simulink model "SimulinkOminidirectinalDrone"  (R2025a)
settings: Solver=ode15s  StartTime=0.0  StopTime=10  RelTol=1e-4
values from neighbouring files (symbols this model uses):
  AUM = 3.057    [Parameter.m]
  Cq = 0.013    [Parameter.m]
  Ct = 0.013    [Parameter.m]
  g = 9.8    [Parameter.m]
  H = 0.05    [Parameter.m]
  Ixx = 0.49827    [Parameter.m]
  Iyy = 0.48993    [Parameter.m]
  Izz = 0.82777    [Parameter.m]
  L = 0.25    [Parameter.m]
  R_rad = 0.15    [Parameter.m]
  rho = 1.18195    [Parameter.m]
  W = diag([0.994, 0.003, 0.003, 0.994, 0.003, 0.003,            0.994, 0.003, 0.003, 0.994, 0.003, 0.003])    [Parameter.m]
libraries: sharedutil x4, aerolibobsolete x1
(part 1 of 2)
settings Model: Creator=Nguyen_Duc  LastModifiedBy=Nguyen_Duc
settings RTWCC: GPUComputeCapability=3.5

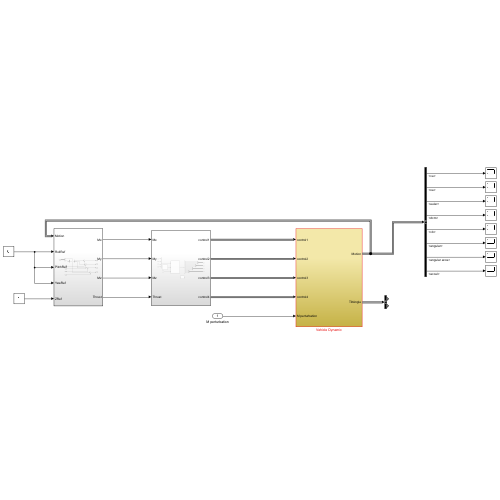
[thumbnail: Simulink's stored preview of the top-level diagram]
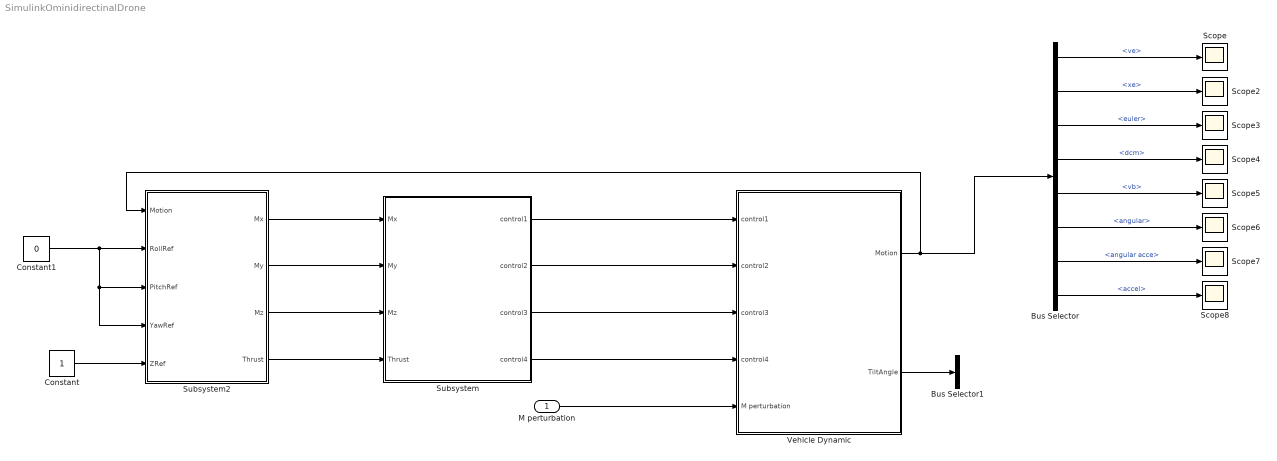
== system SimulinkOminidirectinalDrone ==
  M perturbation : Inport
  Bus Selector : BusSelector  OutputSignals=ve,xe,euler,dcm,vb,angular,angular acce,accel
  Bus Selector1 : BusSelector  OutputSignals=signal1,signal2
  Constant : Constant
  Constant1 : Constant  Value=0
  Scope{,2..8} (8 alike) : Scope
      Scope settings: ActiveDisplayYMinimum=-12.600361564793616  ActiveDisplayYMaximum=158.14211469770717
      Scope2 settings: ActiveDisplayYMinimum=-253.65470239682742  ActiveDisplayYMaximum=2044.3378889341363  DataLoggingVariableName=ScopeData2
      Scope3 settings: ActiveDisplayYMinimum=-3.8093227520417652  ActiveDisplayYMaximum=3.6702175311661223  DataLoggingVariableName=ScopeData3
      Scope4 settings: ActiveDisplayYMinimum=-1.6887966568785009  ActiveDisplayYMaximum=1.3036985575111188  DataLoggingVariableName=ScopeData4
      Scope5 settings: ActiveDisplayYMinimum=-51.9670542151825  ActiveDisplayYMaximum=175.32388672860668  DataLoggingVariableName=ScopeData5
      Scope6 settings: ActiveDisplayYMinimum=-1  ActiveDisplayYMaximum=1  DataLoggingVariableName=ScopeData6
      Scope7 settings: DataLoggingVariableName=ScopeData7
      Scope8 settings: DataLoggingVariableName=ScopeData8
  Subsystem : Subsystem
  Subsystem2 : Subsystem
  Vehicle Dynamic : Subsystem
  wires:
  Subsystem/1(control1) -> Vehicle Dynamic/1(control1)
  Subsystem/2(control2) -> Vehicle Dynamic/2(control2)
  Subsystem/3(control3) -> Vehicle Dynamic/3(control3)
  Subsystem/4(control4) -> Vehicle Dynamic/4(control4)
  M perturbation/1 -> Vehicle Dynamic/5(M perturbation)
  Vehicle Dynamic/2(TiltAngle) -> Bus Selector1/1
  Vehicle Dynamic/1(Motion) -> Bus Selector/1, Subsystem2/1(Motion)
  Bus Selector/1 -> Scope/1  "<ve>"
  Bus Selector/2 -> Scope2/1  "<xe>"
  Bus Selector/3 -> Scope3/1  "<euler>"
  Bus Selector/4 -> Scope4/1  "<dcm>"
  Bus Selector/5 -> Scope5/1  "<vb>"
  Bus Selector/6 -> Scope6/1  "<angular>"
  Bus Selector/7 -> Scope7/1  "<angular acce>"
  Bus Selector/8 -> Scope8/1  "<accel>"
  Constant/1 -> Subsystem2/5(ZRef)
  Constant1/1 -> Subsystem2/4(YawRef), Subsystem2/3(PitchRef), Subsystem2/2(RollRef)
  Subsystem2/1(Mx) -> Subsystem/1(Mx)
  Subsystem2/2(My) -> Subsystem/2(My)
  Subsystem2/3(Mz) -> Subsystem/3(Mz)
  Subsystem2/4(Thrust) -> Subsystem/4(Thrust)

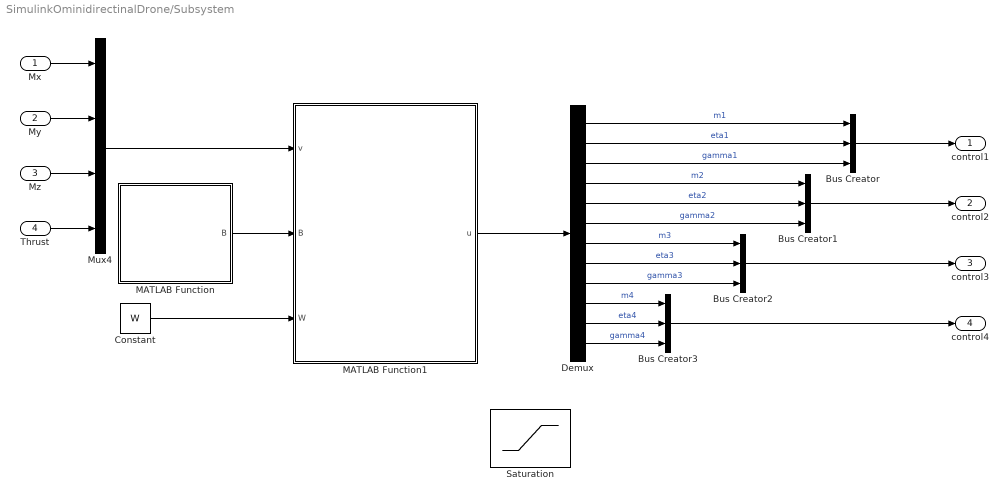
== system SimulinkOminidirectinalDrone/Subsystem ==
  Mx : Inport
  My : Inport  Port=2
  Mz : Inport  Port=3
  Thrust : Inport  Port=4
  Bus Creator{,1..3} (4 alike) : BusCreator  Inputs=3
  Constant : Constant  Value=W
  Demux : Demux  Outputs=12
  MATLAB Function : MATLAB Function  TreatAsAtomicUnit=on
  MATLAB Function1 : MATLAB Function  TreatAsAtomicUnit=on
  Mux4 : Mux
  Saturation : Saturate  UpperLimit="[1  30*pi/180  0.2  1  30*pi/180  0.2  1  30*pi/180  0.2  1  30*pi/180  0.2]"  LowerLimit="[0 -30*pi/180 -0.2  0 -30*pi/180 -0.2  0 -30*pi/180 -0.2  0 -30*pi/180 -0.2]"
  control1 : Outport
  control2 : Outport  Port=2
  control3 : Outport  Port=3
  control4 : Outport  Port=4
  wires:
  MATLAB Function/1(B) -> MATLAB Function1/2(B)
  Mux4/1 -> MATLAB Function1/1(v)
  Demux/1 -> Bus Creator/1  "m1"
  Bus Creator/1 -> control1/1
  Demux/3 -> Bus Creator/3  "gamma1"
  Demux/2 -> Bus Creator/2  "eta1"
  Demux/4 -> Bus Creator1/1  "m2"
  Demux/5 -> Bus Creator1/2  "eta2"
  Demux/6 -> Bus Creator1/3  "gamma2"
  Demux/7 -> Bus Creator2/1  "m3"
  Demux/8 -> Bus Creator2/2  "eta3"
  Demux/9 -> Bus Creator2/3  "gamma3"
  Demux/10 -> Bus Creator3/1  "m4"
  Demux/11 -> Bus Creator3/2  "eta4"
  Demux/12 -> Bus Creator3/3  "gamma4"
  Bus Creator1/1 -> control2/1
  Bus Creator2/1 -> control3/1
  Bus Creator3/1 -> control4/1
  Mx/1 -> Mux4/1
  My/1 -> Mux4/2
  Mz/1 -> Mux4/3
  Thrust/1 -> Mux4/4
  Constant/1 -> MATLAB Function1/3(W)
  MATLAB Function1/1(u) -> Demux/1

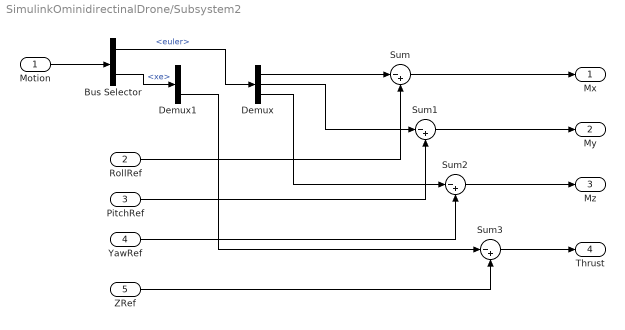
== system SimulinkOminidirectinalDrone/Subsystem2 ==
  Motion : Inport
  RollRef : Inport  Port=2
  PitchRef : Inport  Port=3
  YawRef : Inport  Port=4
  ZRef : Inport  Port=5
  Bus Selector : BusSelector  OutputSignals=euler,xe
  Demux : Demux  Outputs=3
  Demux1 : Demux  Outputs=3
  Sum{,1..3} (4 alike) : Sum  Inputs=|-+
  Mx : Outport
  My : Outport  Port=2
  Mz : Outport  Port=3
  Thrust : Outport  Port=4
  wires:
  Motion/1 -> Bus Selector/1
  Bus Selector/1 -> Demux/1  "<euler>"
  Demux/1 -> Sum/1
  RollRef/1 -> Sum/2
  Sum/1 -> Mx/1
  PitchRef/1 -> Sum1/2
  Sum1/1 -> My/1
  Demux/2 -> Sum1/1
  Sum2/1 -> Mz/1
  Demux/3 -> Sum2/1
  YawRef/1 -> Sum2/2
  Bus Selector/2 -> Demux1/1  "<xe>"
  Sum3/1 -> Thrust/1
  Demux1/3 -> Sum3/1
  ZRef/1 -> Sum3/2

== system SimulinkOminidirectinalDrone/Vehicle Dynamic ==
  control1 : Inport
  control2 : Inport  Port=2
  control3 : Inport  Port=3
  control4 : Inport  Port=4
  M perturbation : Inport  Port=5
  6DOF (Euler Angles) : aerolibobsolete/6DOF (Euler Angles)  units=Metric (MKS)  mtype=Fixed  rep=Euler Angles  xme_0=[0 0 0]  Vm_0=[0 0 0]  eul_0=[0 0 0]  pm_0=[0 0 0]  mass_0=AUM  mass_e=0.5  mass_f=2.0  inertia=[0.49827 0 0; 0 0.48993 0; 0 0 0.82777]  inertia_e=eye(3)  inertia_f=2*eye(3)  k_quat=1.0  vre_flag=on  abi_flag=off  aMode=0  xme_statename=''  Vm_statename=''  eul_statename=''  quat_statename=''  pm_statename=''  mass_statename=''
  Bus Creator : BusCreator  Inputs=8
  Constant : Constant  Value=[0 0 g*AUM]'
  Matrix Multiply : Product  Multiplication=Matrix(*)
  Subsystem1 : Subsystem
  Sum : Sum  Inputs=++|
  Sum1 : Sum  Inputs=|++
  actuator : Subsystem
  Motion : Outport
  TiltAngle : Outport  Port=2
  wires:
  control3/1 -> actuator/4(control3)
  M perturbation/1 -> Sum1/2
  Matrix Multiply/1 -> Sum/1
  6DOF (Euler Angles)/7 -> Bus Creator/7, Subsystem1/2(omegadot)  "angular acce"
  6DOF (Euler Angles)/3 -> Bus Creator/3  "euler"
  Bus Creator/1 -> Motion/1
  control1/1 -> actuator/2(control1)
  6DOF (Euler Angles)/2 -> Bus Creator/2  "xe"
  6DOF (Euler Angles)/1 -> Bus Creator/1  "ve"
  control2/1 -> actuator/3(control2)
  control4/1 -> actuator/5(control4)
  Constant/1 -> Matrix Multiply/2
  6DOF (Euler Angles)/8 -> Bus Creator/8  "accel"
  6DOF (Euler Angles)/6 -> Subsystem1/1(omega), Bus Creator/6  "angular"
  6DOF (Euler Angles)/5 -> Bus Creator/5  "vb"
  6DOF (Euler Angles)/4 -> Matrix Multiply/1, Bus Creator/4  "dcm"
  actuator/3(TiltAngle) -> TiltAngle/1
  Subsystem1/1(Rotation) -> actuator/1(rotation)
  Sum/1 -> 6DOF (Euler Angles)/1
  actuator/1(Forces) -> Sum/2
  actuator/2(Moments) -> Sum1/1
  Sum1/1 -> 6DOF (Euler Angles)/2

== system SimulinkOminidirectinalDrone/Vehicle Dynamic/Subsystem1 ==
  omega : Inport
  omegadot : Inport  Port=2
  Bus Creator : BusCreator  Inputs=6
  Delay : Delay
  Delay1 : Delay
  Delay2 : Delay
  Demux : Demux  Outputs=3
  Demux1 : Demux  Outputs=3
  Rotation : Outport
  wires:
  omega/1 -> Demux/1
  omegadot/1 -> Demux1/1
  Bus Creator/1 -> Rotation/1
  Demux/1 -> Bus Creator/1  "p"
  Demux/2 -> Bus Creator/2  "q"
  Demux/3 -> Bus Creator/3  "r"
  Delay/1 -> Bus Creator/4  "pdot"
  Delay2/1 -> Bus Creator/6  "rdot"
  Delay1/1 -> Bus Creator/5  "qdot"
  Demux1/1 -> Delay/1  "pdot"
  Demux1/2 -> Delay1/1  "qdot"
  Demux1/3 -> Delay2/1  "rdot"

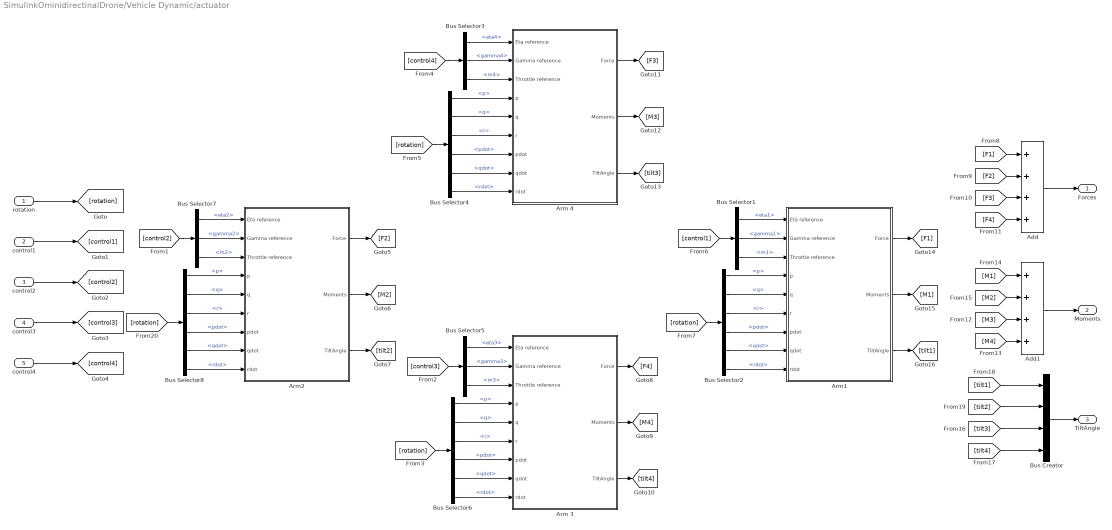
== system SimulinkOminidirectinalDrone/Vehicle Dynamic/actuator ==
  rotation : Inport
  control1 : Inport  Port=2
  control2 : Inport  Port=3
  control3 : Inport  Port=4
  control4 : Inport  Port=5
  Add : Sum  Inputs=++++
  Add1 : Sum  Inputs=++++
  Arm 3 : Subsystem
  Arm 4 : Subsystem
  Arm1 : Subsystem
  Arm2 : Subsystem
  Bus Creator : BusCreator  Inputs=4
  Bus Selector1 : BusSelector  OutputSignals=eta1,gamma1,m1
  Bus Selector{2,4,6,8} (4 alike) : BusSelector  OutputSignals=p,q,r,pdot,qdot,rdot
  Bus Selector3 : BusSelector  OutputSignals=eta4,gamma4,m4
  Bus Selector5 : BusSelector  OutputSignals=eta3,gamma3,m3
  Bus Selector7 : BusSelector  OutputSignals=eta2,gamma2,m2
  Forces : Outport
  Moments : Outport  Port=2
  TiltAngle : Outport  Port=3
  wires:
  control3/1 -> [control3]
  Add/1 -> Forces/1
  [F4] -> Add/4
  Arm1/3(TiltAngle) -> [tilt1]
  [M3] -> Add1/3
  [control1] -> Bus Selector1/1
  Arm1/2(Moments) -> [M1]
  Arm 4/1(Force) -> [F3]
  Bus Selector2/3 -> Arm1/6(r)  "<r>"
  [M2] -> Add1/2
  Arm2/1(Force) -> [F2]
  Arm1/1(Force) -> [F1]
  [M1] -> Add1/1
  [M4] -> Add1/4
  Add1/1 -> Moments/1
  Arm 3/1(Force) -> [F4]
  Bus Selector2/2 -> Arm1/5(q)  "<q>"
  Arm 4/2(Moments) -> [M3]
  Arm 3/2(Moments) -> [M4]
  control1/1 -> [control1]
  Arm2/3(TiltAngle) -> [tilt2]
  Arm 3/3(TiltAngle) -> [tilt4]
  control2/1 -> [control2]
  Bus Selector2/1 -> Arm1/4(p)  "<p>"
  Arm2/2(Moments) -> [M2]
  Arm 4/3(TiltAngle) -> [tilt3]
  rotation/1 -> [rotation]
  control4/1 -> [control4]
  [F3] -> Add/3
  [F1] -> Add/1
  [F2] -> Add/2
  [tilt1] -> Bus Creator/1
  [tilt2] -> Bus Creator/2
  [tilt3] -> Bus Creator/3
  [tilt4] -> Bus Creator/4
  Bus Creator/1 -> TiltAngle/1
  [rotation] -> Bus Selector2/1
  Bus Selector1/1 -> Arm1/1(Eta reference)  "<eta1>"
  Bus Selector1/2 -> Arm1/2(Gamma reference)  "<gamma1>"
  Bus Selector1/3 -> Arm1/3(Throttle reference)  "<m1>"
  Bus Selector2/4 -> Arm1/7(pdot)  "<pdot>"
  [control4] -> Bus Selector3/1
  [control3] -> Bus Selector5/1
  [control2] -> Bus Selector7/1
  Bus Selector3/1 -> Arm 4/1(Eta reference)  "<eta4>"
  Bus Selector3/2 -> Arm 4/2(Gamma reference)  "<gamma4>"
  Bus Selector3/3 -> Arm 4/3(Throttle reference)  "<m4>"
  Bus Selector5/1 -> Arm 3/1(Eta reference)  "<eta3>"
  Bus Selector5/2 -> Arm 3/2(Gamma reference)  "<gamma3>"
  Bus Selector5/3 -> Arm 3/3(Throttle reference)  "<m3>"
  Bus Selector7/1 -> Arm2/1(Eta reference)  "<eta2>"
  Bus Selector7/2 -> Arm2/2(Gamma reference)  "<gamma2>"
  Bus Selector7/3 -> Arm2/3(Throttle reference)  "<m2>"
  Bus Selector2/5 -> Arm1/8(qdot)  "<qdot>"
  Bus Selector2/6 -> Arm1/9(rdot)  "<rdot>"
  Bus Selector6/1 -> Arm 3/4(p)  "<p>"
  Bus Selector6/2 -> Arm 3/5(q)  "<q>"
  [rotation] -> Bus Selector6/1
  Bus Selector6/3 -> Arm 3/6(r)  "<r>"
  Bus Selector6/5 -> Arm 3/8(qdot)  "<qdot>"
  Bus Selector6/4 -> Arm 3/7(pdot)  "<pdot>"
  Bus Selector6/6 -> Arm 3/9(rdot)  "<rdot>"
  Bus Selector8/1 -> Arm2/4(p)  "<p>"
  Bus Selector8/2 -> Arm2/5(q)  "<q>"
  [rotation] -> Bus Selector8/1
  Bus Selector8/3 -> Arm2/6(r)  "<r>"
  Bus Selector8/5 -> Arm2/8(qdot)  "<qdot>"
  Bus Selector8/4 -> Arm2/7(pdot)  "<pdot>"
  Bus Selector8/6 -> Arm2/9(rdot)  "<rdot>"
  Bus Selector4/1 -> Arm 4/4(p)  "<p>"
  Bus Selector4/2 -> Arm 4/5(q)  "<q>"
  [rotation] -> Bus Selector4/1
  Bus Selector4/3 -> Arm 4/6(r)  "<r>"
  Bus Selector4/5 -> Arm 4/8(qdot)  "<qdot>"
  Bus Selector4/4 -> Arm 4/7(pdot)  "<pdot>"
  Bus Selector4/6 -> Arm 4/9(rdot)  "<rdot>"

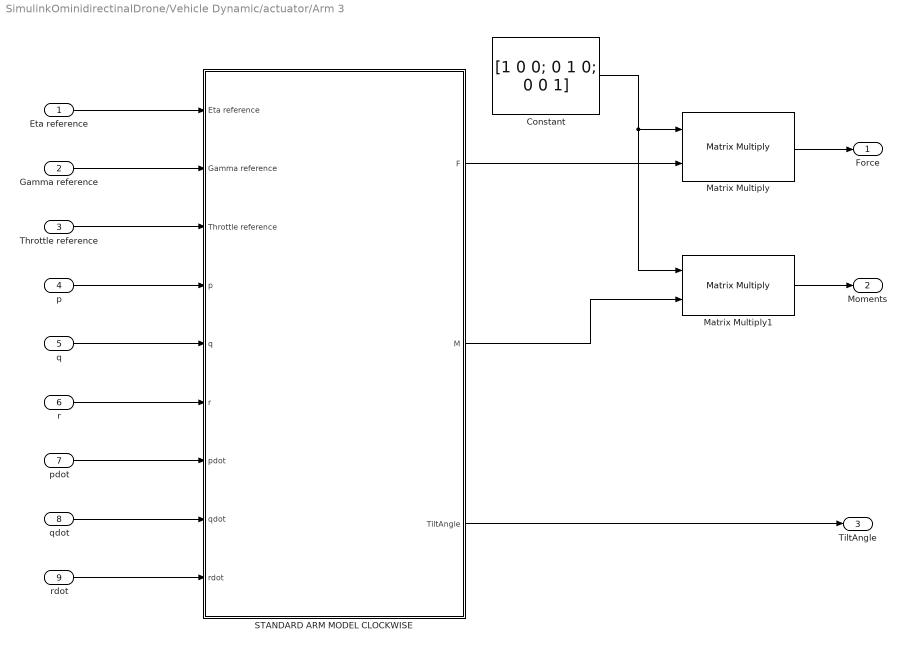
== system SimulinkOminidirectinalDrone/Vehicle Dynamic/actuator/Arm 3 ==
  Eta reference : Inport
  Gamma reference : Inport  Port=2
  Throttle reference : Inport  Port=3
  p : Inport  Port=4
  q : Inport  Port=5
  r : Inport  Port=6
  pdot : Inport  Port=7
  qdot : Inport  Port=8
  rdot : Inport  Port=9
  Constant : Constant  Value=[1 0 0; 0 1 0; 0 0 1]
  Matrix Multiply : Product  Multiplication=Matrix(*)
  Matrix Multiply1 : Product  Multiplication=Matrix(*)
  STANDARD ARM MODEL CLOCKWISE : Subsystem
  Force : Outport
  Moments : Outport  Port=2
  TiltAngle : Outport  Port=3
  wires:
  Gamma reference/1 -> STANDARD ARM MODEL CLOCKWISE/2(Gamma reference)
  Eta reference/1 -> STANDARD ARM MODEL CLOCKWISE/1(Eta reference)
  Matrix Multiply1/1 -> Moments/1
  STANDARD ARM MODEL CLOCKWISE/1(F) -> Matrix Multiply/2
  Throttle reference/1 -> STANDARD ARM MODEL CLOCKWISE/3(Throttle reference)
  r/1 -> STANDARD ARM MODEL CLOCKWISE/6(r)
  p/1 -> STANDARD ARM MODEL CLOCKWISE/4(p)
  q/1 -> STANDARD ARM MODEL CLOCKWISE/5(q)
  STANDARD ARM MODEL CLOCKWISE/2(M) -> Matrix Multiply1/2
  pdot/1 -> STANDARD ARM MODEL CLOCKWISE/7(pdot)
  qdot/1 -> STANDARD ARM MODEL CLOCKWISE/8(qdot)
  rdot/1 -> STANDARD ARM MODEL CLOCKWISE/9(rdot)
  Constant/1 -> Matrix Multiply1/1, Matrix Multiply/1
  Matrix Multiply/1 -> Force/1
  STANDARD ARM MODEL CLOCKWISE/3(TiltAngle) -> TiltAngle/1

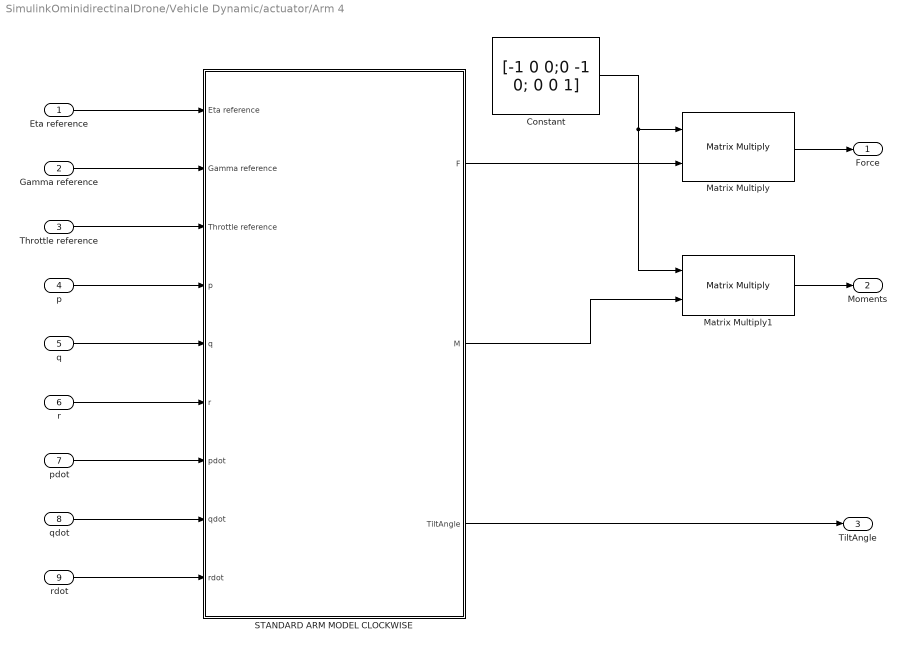
== system SimulinkOminidirectinalDrone/Vehicle Dynamic/actuator/Arm 4 ==
  Eta reference : Inport
  Gamma reference : Inport  Port=2
  Throttle reference : Inport  Port=3
  p : Inport  Port=4
  q : Inport  Port=5
  r : Inport  Port=6
  pdot : Inport  Port=7
  qdot : Inport  Port=8
  rdot : Inport  Port=9
  Constant : Constant  Value=[-1 0 0;0 -1 0; 0 0 1]
  Matrix Multiply : Product  Multiplication=Matrix(*)
  Matrix Multiply1 : Product  Multiplication=Matrix(*)
  STANDARD ARM MODEL CLOCKWISE : Subsystem
  Force : Outport
  Moments : Outport  Port=2
  TiltAngle : Outport  Port=3
  wires:
  Gamma reference/1 -> STANDARD ARM MODEL CLOCKWISE/2(Gamma reference)
  Eta reference/1 -> STANDARD ARM MODEL CLOCKWISE/1(Eta reference)
  Matrix Multiply1/1 -> Moments/1
  STANDARD ARM MODEL CLOCKWISE/1(F) -> Matrix Multiply/2
  Throttle reference/1 -> STANDARD ARM MODEL CLOCKWISE/3(Throttle reference)
  r/1 -> STANDARD ARM MODEL CLOCKWISE/6(r)
  p/1 -> STANDARD ARM MODEL CLOCKWISE/4(p)
  q/1 -> STANDARD ARM MODEL CLOCKWISE/5(q)
  STANDARD ARM MODEL CLOCKWISE/2(M) -> Matrix Multiply1/2
  pdot/1 -> STANDARD ARM MODEL CLOCKWISE/7(pdot)
  qdot/1 -> STANDARD ARM MODEL CLOCKWISE/8(qdot)
  rdot/1 -> STANDARD ARM MODEL CLOCKWISE/9(rdot)
  Constant/1 -> Matrix Multiply1/1, Matrix Multiply/1
  Matrix Multiply/1 -> Force/1
  STANDARD ARM MODEL CLOCKWISE/3(TiltAngle) -> TiltAngle/1

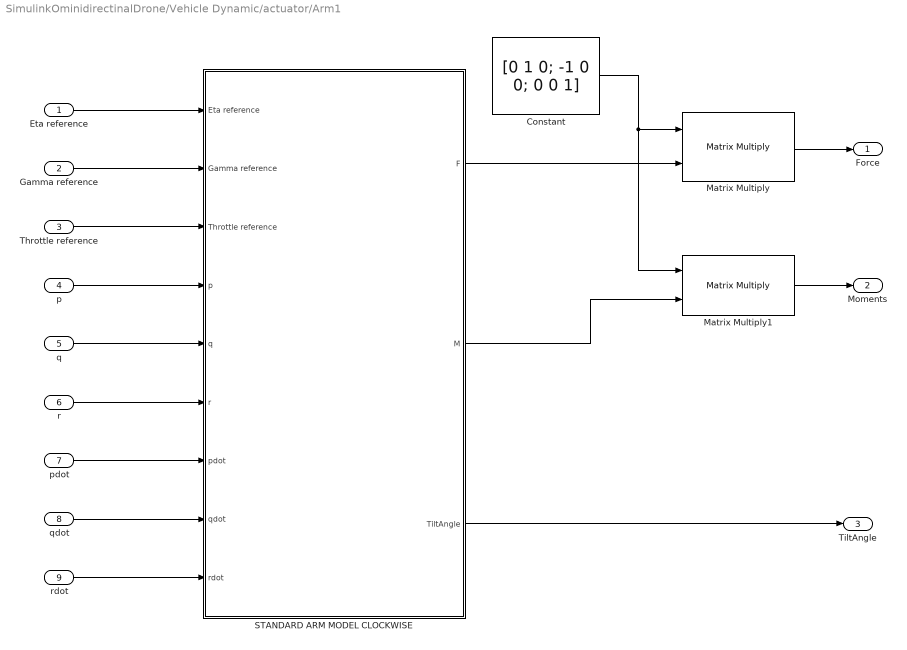
== system SimulinkOminidirectinalDrone/Vehicle Dynamic/actuator/Arm1 ==
  Eta reference : Inport
  Gamma reference : Inport  Port=2
  Throttle reference : Inport  Port=3
  p : Inport  Port=4
  q : Inport  Port=5
  r : Inport  Port=6
  pdot : Inport  Port=7
  qdot : Inport  Port=8
  rdot : Inport  Port=9
  Constant : Constant  Value=[0 1 0; -1 0 0; 0 0 1]
  Matrix Multiply : Product  Multiplication=Matrix(*)
  Matrix Multiply1 : Product  Multiplication=Matrix(*)
  STANDARD ARM MODEL CLOCKWISE : Subsystem
  Force : Outport
  Moments : Outport  Port=2
  TiltAngle : Outport  Port=3
  wires:
  Gamma reference/1 -> STANDARD ARM MODEL CLOCKWISE/2(Gamma reference)
  Eta reference/1 -> STANDARD ARM MODEL CLOCKWISE/1(Eta reference)
  Matrix Multiply1/1 -> Moments/1
  STANDARD ARM MODEL CLOCKWISE/1(F) -> Matrix Multiply/2
  Throttle reference/1 -> STANDARD ARM MODEL CLOCKWISE/3(Throttle reference)
  r/1 -> STANDARD ARM MODEL CLOCKWISE/6(r)
  p/1 -> STANDARD ARM MODEL CLOCKWISE/4(p)
  q/1 -> STANDARD ARM MODEL CLOCKWISE/5(q)
  STANDARD ARM MODEL CLOCKWISE/2(M) -> Matrix Multiply1/2
  pdot/1 -> STANDARD ARM MODEL CLOCKWISE/7(pdot)
  qdot/1 -> STANDARD ARM MODEL CLOCKWISE/8(qdot)
  rdot/1 -> STANDARD ARM MODEL CLOCKWISE/9(rdot)
  Constant/1 -> Matrix Multiply1/1, Matrix Multiply/1
  Matrix Multiply/1 -> Force/1
  STANDARD ARM MODEL CLOCKWISE/3(TiltAngle) -> TiltAngle/1

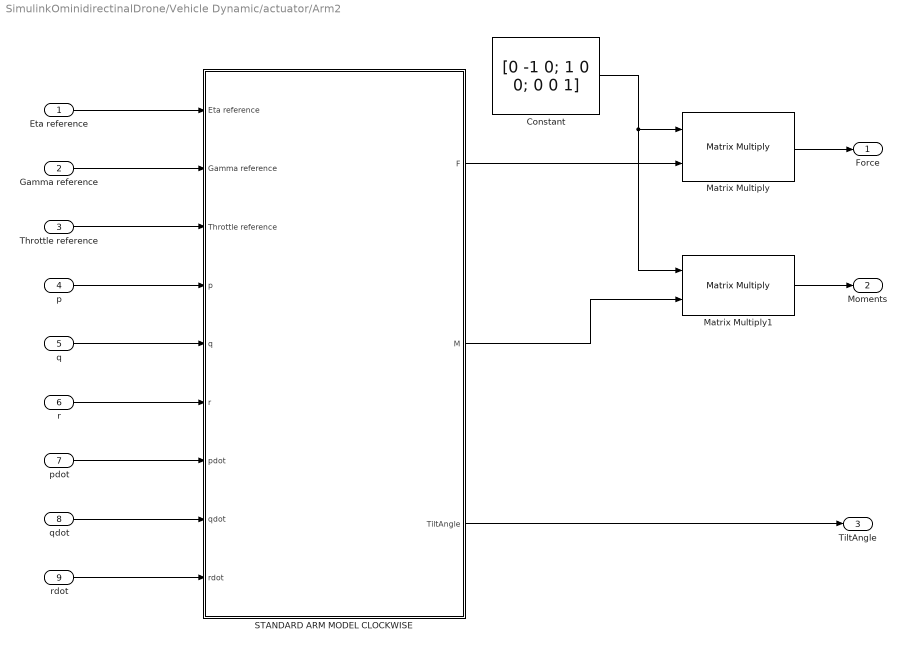
== system SimulinkOminidirectinalDrone/Vehicle Dynamic/actuator/Arm2 ==
  Eta reference : Inport
  Gamma reference : Inport  Port=2
  Throttle reference : Inport  Port=3
  p : Inport  Port=4
  q : Inport  Port=5
  r : Inport  Port=6
  pdot : Inport  Port=7
  qdot : Inport  Port=8
  rdot : Inport  Port=9
  Constant : Constant  Value=[0 -1 0; 1 0 0; 0 0 1]
  Matrix Multiply : Product  Multiplication=Matrix(*)
  Matrix Multiply1 : Product  Multiplication=Matrix(*)
  STANDARD ARM MODEL CLOCKWISE : Subsystem
  Force : Outport
  Moments : Outport  Port=2
  TiltAngle : Outport  Port=3
  wires:
  Gamma reference/1 -> STANDARD ARM MODEL CLOCKWISE/2(Gamma reference)
  Eta reference/1 -> STANDARD ARM MODEL CLOCKWISE/1(Eta reference)
  Matrix Multiply1/1 -> Moments/1
  STANDARD ARM MODEL CLOCKWISE/1(F) -> Matrix Multiply/2
  Throttle reference/1 -> STANDARD ARM MODEL CLOCKWISE/3(Throttle reference)
  r/1 -> STANDARD ARM MODEL CLOCKWISE/6(r)
  p/1 -> STANDARD ARM MODEL CLOCKWISE/4(p)
  q/1 -> STANDARD ARM MODEL CLOCKWISE/5(q)
  STANDARD ARM MODEL CLOCKWISE/2(M) -> Matrix Multiply1/2
  pdot/1 -> STANDARD ARM MODEL CLOCKWISE/7(pdot)
  qdot/1 -> STANDARD ARM MODEL CLOCKWISE/8(qdot)
  rdot/1 -> STANDARD ARM MODEL CLOCKWISE/9(rdot)
  Constant/1 -> Matrix Multiply1/1, Matrix Multiply/1
  Matrix Multiply/1 -> Force/1
  STANDARD ARM MODEL CLOCKWISE/3(TiltAngle) -> TiltAngle/1

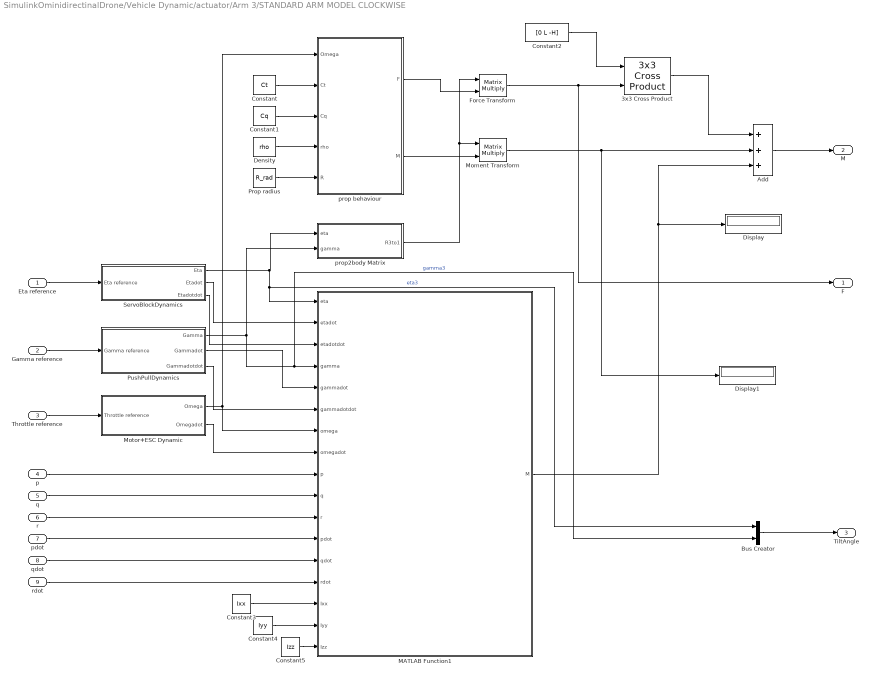
== system SimulinkOminidirectinalDrone/Vehicle Dynamic/actuator/Arm 3/STANDARD ARM MODEL CLOCKWISE ==
  Eta reference : Inport
  Gamma reference : Inport  Port=2
  Throttle reference : Inport  Port=3
  p : Inport  Port=4
  q : Inport  Port=5
  r : Inport  Port=6
  pdot : Inport  Port=7
  qdot : Inport  Port=8
  rdot : Inport  Port=9
  3x3 Cross Product : sharedutil/3x3 Cross Product  aMode=aMode
      settings: LibrarySourceBlock=aerolibutil/3x3 Cross Product
  Add : Sum  Inputs=+++
  Bus Creator : BusCreator  Inputs=2
  Constant : Constant  Value=Ct
  Constant1 : Constant  Value=Cq
  Constant2 : Constant  Value=[0 L -H]
  Constant3 : Constant  Value=Ixx
  Constant4 : Constant  Value=Iyy
  Constant5 : Constant  Value=Izz
  Density : Constant  Value=rho
  Display : Display
  Display1 : Display
  Force Transform : Product  Multiplication=Matrix(*)
  MATLAB Function1 : MATLAB Function  TreatAsAtomicUnit=on
  Moment Transform : Product  Multiplication=Matrix(*)
  Motor+ESC Dynamic : Subsystem
  Prop radius : Constant  Value=R_rad
  PushPullDynamics : Subsystem
  ServoBlockDynamics : Subsystem
  prop behaviour : MATLAB Function  TreatAsAtomicUnit=on
  prop2body Matrix : MATLAB Function  TreatAsAtomicUnit=on
  F : Outport
  M : Outport  Port=2
  TiltAngle : Outport  Port=3
  wires:
  Motor+ESC Dynamic/2(Omegadot) -> MATLAB Function1/8(omegadot)
  PushPullDynamics/3(Gammadotdot) -> MATLAB Function1/6(gammadotdot)
  Constant5/1 -> MATLAB Function1/17(Izz)
  Constant4/1 -> MATLAB Function1/16(Iyy)
  p/1 -> MATLAB Function1/9(p)
  prop2body Matrix/1(R3to1) -> Moment Transform/1, Force Transform/1
  Moment Transform/1 -> Display1/1, Add/2
  Prop radius/1 -> prop behaviour/5(R)
  Gamma reference/1 -> PushPullDynamics/1(Gamma reference)
  qdot/1 -> MATLAB Function1/13(qdot)
  Constant1/1 -> prop behaviour/3(Cq)
  Throttle reference/1 -> Motor+ESC Dynamic/1(Throttle reference)
  3x3 Cross Product/1 -> Add/1
  q/1 -> MATLAB Function1/10(q)
  Density/1 -> prop behaviour/4(rho)
  Motor+ESC Dynamic/1(Omega) -> MATLAB Function1/7(omega), prop behaviour/1(Omega)
  ServoBlockDynamics/3(Etadotdot) -> MATLAB Function1/3(etadotdot)
  prop behaviour/2(M) -> Moment Transform/2
  Constant3/1 -> MATLAB Function1/15(Ixx)
  PushPullDynamics/1(Gamma) -> Bus Creator/2, MATLAB Function1/4(gamma), prop2body Matrix/2(gamma)  "gamma3"
  Constant2/1 -> 3x3 Cross Product/1
  Force Transform/1 -> F/1, 3x3 Cross Product/2
  MATLAB Function1/1(M) -> Display/1, Add/3
  ServoBlockDynamics/1(Eta) -> Bus Creator/1, MATLAB Function1/1(eta), prop2body Matrix/1(eta)  "eta3"
  r/1 -> MATLAB Function1/11(r)
  rdot/1 -> MATLAB Function1/14(rdot)
  Eta reference/1 -> ServoBlockDynamics/1(Eta reference)
  Bus Creator/1 -> TiltAngle/1
  PushPullDynamics/2(Gammadot) -> MATLAB Function1/5(gammadot)
  pdot/1 -> MATLAB Function1/12(pdot)
  prop behaviour/1(F) -> Force Transform/2
  Constant/1 -> prop behaviour/2(Ct)
  Add/1 -> M/1
  ServoBlockDynamics/2(Etadot) -> MATLAB Function1/2(etadot)

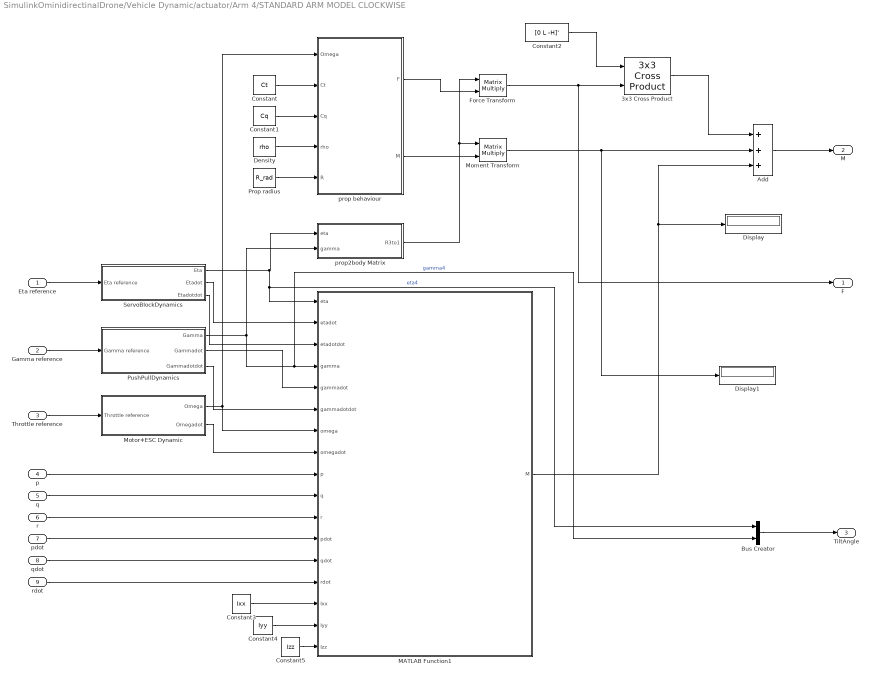
== system SimulinkOminidirectinalDrone/Vehicle Dynamic/actuator/Arm 4/STANDARD ARM MODEL CLOCKWISE ==
  Eta reference : Inport
  Gamma reference : Inport  Port=2
  Throttle reference : Inport  Port=3
  p : Inport  Port=4
  q : Inport  Port=5
  r : Inport  Port=6
  pdot : Inport  Port=7
  qdot : Inport  Port=8
  rdot : Inport  Port=9
  3x3 Cross Product : sharedutil/3x3 Cross Product  aMode=aMode
      settings: LibrarySourceBlock=aerolibutil/3x3 Cross Product
  Add : Sum  Inputs=+++
  Bus Creator : BusCreator  Inputs=2
  Constant : Constant  Value=Ct
  Constant1 : Constant  Value=Cq
  Constant2 : Constant  Value=[0 L -H]'
  Constant3 : Constant  Value=Ixx
  Constant4 : Constant  Value=Iyy
  Constant5 : Constant  Value=Izz
  Density : Constant  Value=rho
  Display : Display
  Display1 : Display
  Force Transform : Product  Multiplication=Matrix(*)
  MATLAB Function1 : MATLAB Function  TreatAsAtomicUnit=on
  Moment Transform : Product  Multiplication=Matrix(*)
  Motor+ESC Dynamic : Subsystem
  Prop radius : Constant  Value=R_rad
  PushPullDynamics : Subsystem
  ServoBlockDynamics : Subsystem
  prop behaviour : MATLAB Function  TreatAsAtomicUnit=on
  prop2body Matrix : MATLAB Function  TreatAsAtomicUnit=on
  F : Outport
  M : Outport  Port=2
  TiltAngle : Outport  Port=3
  wires:
  Motor+ESC Dynamic/2(Omegadot) -> MATLAB Function1/8(omegadot)
  PushPullDynamics/3(Gammadotdot) -> MATLAB Function1/6(gammadotdot)
  Constant5/1 -> MATLAB Function1/17(Izz)
  Constant4/1 -> MATLAB Function1/16(Iyy)
  p/1 -> MATLAB Function1/9(p)
  prop2body Matrix/1(R3to1) -> Moment Transform/1, Force Transform/1
  Moment Transform/1 -> Display1/1, Add/2
  Prop radius/1 -> prop behaviour/5(R)
  Gamma reference/1 -> PushPullDynamics/1(Gamma reference)
  qdot/1 -> MATLAB Function1/13(qdot)
  Constant1/1 -> prop behaviour/3(Cq)
  Throttle reference/1 -> Motor+ESC Dynamic/1(Throttle reference)
  3x3 Cross Product/1 -> Add/1
  q/1 -> MATLAB Function1/10(q)
  Density/1 -> prop behaviour/4(rho)
  Motor+ESC Dynamic/1(Omega) -> MATLAB Function1/7(omega), prop behaviour/1(Omega)
  ServoBlockDynamics/3(Etadotdot) -> MATLAB Function1/3(etadotdot)
  prop behaviour/2(M) -> Moment Transform/2
  Constant3/1 -> MATLAB Function1/15(Ixx)
  PushPullDynamics/1(Gamma) -> Bus Creator/2, MATLAB Function1/4(gamma), prop2body Matrix/2(gamma)  "gamma4"
  Constant2/1 -> 3x3 Cross Product/1
  Force Transform/1 -> F/1, 3x3 Cross Product/2
  MATLAB Function1/1(M) -> Display/1, Add/3
  ServoBlockDynamics/1(Eta) -> Bus Creator/1, MATLAB Function1/1(eta), prop2body Matrix/1(eta)  "eta4"
  r/1 -> MATLAB Function1/11(r)
  rdot/1 -> MATLAB Function1/14(rdot)
  Eta reference/1 -> ServoBlockDynamics/1(Eta reference)
  Bus Creator/1 -> TiltAngle/1
  PushPullDynamics/2(Gammadot) -> MATLAB Function1/5(gammadot)
  pdot/1 -> MATLAB Function1/12(pdot)
  prop behaviour/1(F) -> Force Transform/2
  Constant/1 -> prop behaviour/2(Ct)
  Add/1 -> M/1
  ServoBlockDynamics/2(Etadot) -> MATLAB Function1/2(etadot)

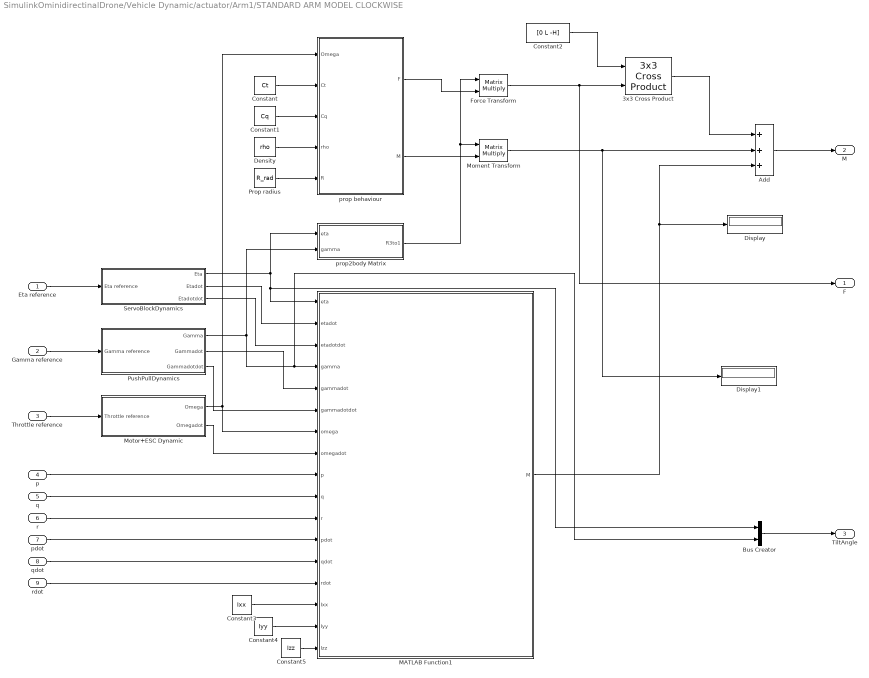
== system SimulinkOminidirectinalDrone/Vehicle Dynamic/actuator/Arm1/STANDARD ARM MODEL CLOCKWISE ==
  Eta reference : Inport
  Gamma reference : Inport  Port=2
  Throttle reference : Inport  Port=3
  p : Inport  Port=4
  q : Inport  Port=5
  r : Inport  Port=6
  pdot : Inport  Port=7
  qdot : Inport  Port=8
  rdot : Inport  Port=9
  3x3 Cross Product : sharedutil/3x3 Cross Product  aMode=aMode
      settings: LibrarySourceBlock=aerolibutil/3x3 Cross Product
  Add : Sum  Inputs=+++
  Bus Creator : BusCreator  Inputs=2
  Constant : Constant  Value=Ct
  Constant1 : Constant  Value=Cq
  Constant2 : Constant  Value=[0 L -H]
  Constant3 : Constant  Value=Ixx
  Constant4 : Constant  Value=Iyy
  Constant5 : Constant  Value=Izz
  Density : Constant  Value=rho
  Display : Display
  Display1 : Display
  Force Transform : Product  Multiplication=Matrix(*)
  MATLAB Function1 : MATLAB Function  TreatAsAtomicUnit=on
  Moment Transform : Product  Multiplication=Matrix(*)
  Motor+ESC Dynamic : Subsystem
  Prop radius : Constant  Value=R_rad
  PushPullDynamics : Subsystem
  ServoBlockDynamics : Subsystem
  prop behaviour : MATLAB Function  TreatAsAtomicUnit=on
  prop2body Matrix : MATLAB Function  TreatAsAtomicUnit=on
  F : Outport
  M : Outport  Port=2
  TiltAngle : Outport  Port=3
  wires:
  Motor+ESC Dynamic/2(Omegadot) -> MATLAB Function1/8(omegadot)
  PushPullDynamics/3(Gammadotdot) -> MATLAB Function1/6(gammadotdot)
  Constant5/1 -> MATLAB Function1/17(Izz)
  Constant4/1 -> MATLAB Function1/16(Iyy)
  p/1 -> MATLAB Function1/9(p)
  prop2body Matrix/1(R3to1) -> Moment Transform/1, Force Transform/1
  Moment Transform/1 -> Display1/1, Add/2
  Prop radius/1 -> prop behaviour/5(R)
  Gamma reference/1 -> PushPullDynamics/1(Gamma reference)
  qdot/1 -> MATLAB Function1/13(qdot)
  Constant1/1 -> prop behaviour/3(Cq)
  Throttle reference/1 -> Motor+ESC Dynamic/1(Throttle reference)
  3x3 Cross Product/1 -> Add/1
  q/1 -> MATLAB Function1/10(q)
  Density/1 -> prop behaviour/4(rho)
  Motor+ESC Dynamic/1(Omega) -> MATLAB Function1/7(omega), prop behaviour/1(Omega)
  ServoBlockDynamics/3(Etadotdot) -> MATLAB Function1/3(etadotdot)
  prop behaviour/2(M) -> Moment Transform/2
  Constant3/1 -> MATLAB Function1/15(Ixx)
  PushPullDynamics/1(Gamma) -> Bus Creator/2, MATLAB Function1/4(gamma), prop2body Matrix/2(gamma)
  Constant2/1 -> 3x3 Cross Product/1
  Force Transform/1 -> F/1, 3x3 Cross Product/2
  MATLAB Function1/1(M) -> Display/1, Add/3
  ServoBlockDynamics/1(Eta) -> prop2body Matrix/1(eta), Bus Creator/1, MATLAB Function1/1(eta)
  r/1 -> MATLAB Function1/11(r)
  rdot/1 -> MATLAB Function1/14(rdot)
  Eta reference/1 -> ServoBlockDynamics/1(Eta reference)
  Bus Creator/1 -> TiltAngle/1
  PushPullDynamics/2(Gammadot) -> MATLAB Function1/5(gammadot)
  pdot/1 -> MATLAB Function1/12(pdot)
  prop behaviour/1(F) -> Force Transform/2
  Constant/1 -> prop behaviour/2(Ct)
  Add/1 -> M/1
  ServoBlockDynamics/2(Etadot) -> MATLAB Function1/2(etadot)

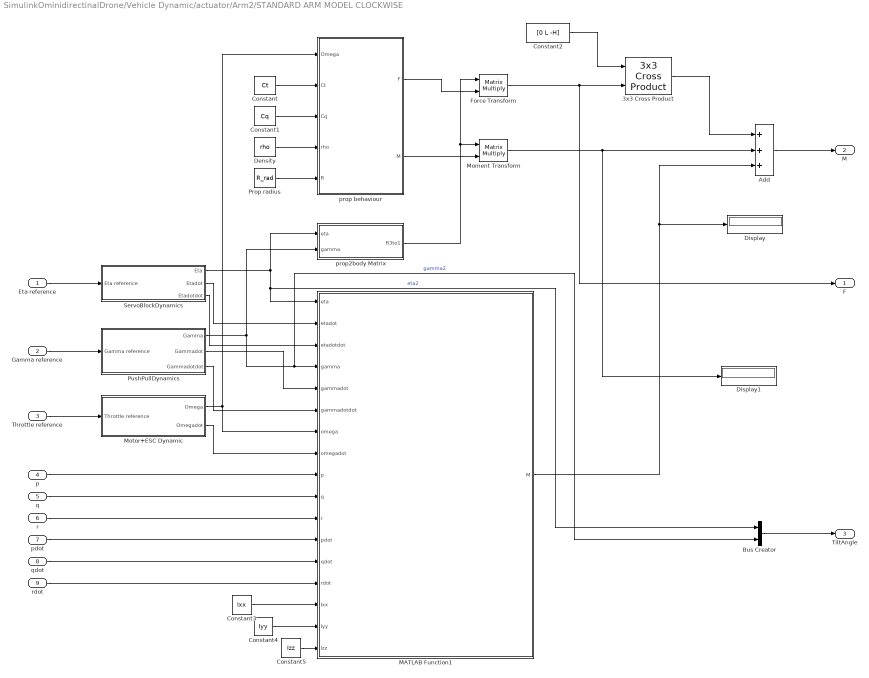
== system SimulinkOminidirectinalDrone/Vehicle Dynamic/actuator/Arm2/STANDARD ARM MODEL CLOCKWISE ==
  Eta reference : Inport
  Gamma reference : Inport  Port=2
  Throttle reference : Inport  Port=3
  p : Inport  Port=4
  q : Inport  Port=5
  r : Inport  Port=6
  pdot : Inport  Port=7
  qdot : Inport  Port=8
  rdot : Inport  Port=9
  3x3 Cross Product : sharedutil/3x3 Cross Product  aMode=aMode
      settings: LibrarySourceBlock=aerolibutil/3x3 Cross Product
  Add : Sum  Inputs=+++
  Bus Creator : BusCreator  Inputs=2
  Constant : Constant  Value=Ct
  Constant1 : Constant  Value=Cq
  Constant2 : Constant  Value=[0 L -H]
  Constant3 : Constant  Value=Ixx
  Constant4 : Constant  Value=Iyy
  Constant5 : Constant  Value=Izz
  Density : Constant  Value=rho
  Display : Display
  Display1 : Display
  Force Transform : Product  Multiplication=Matrix(*)
  MATLAB Function1 : MATLAB Function  TreatAsAtomicUnit=on
  Moment Transform : Product  Multiplication=Matrix(*)
  Motor+ESC Dynamic : Subsystem
  Prop radius : Constant  Value=R_rad
  PushPullDynamics : Subsystem
  ServoBlockDynamics : Subsystem
  prop behaviour : MATLAB Function  TreatAsAtomicUnit=on
  prop2body Matrix : MATLAB Function  TreatAsAtomicUnit=on
  F : Outport
  M : Outport  Port=2
  TiltAngle : Outport  Port=3
  wires:
  Motor+ESC Dynamic/2(Omegadot) -> MATLAB Function1/8(omegadot)
  PushPullDynamics/3(Gammadotdot) -> MATLAB Function1/6(gammadotdot)
  Constant5/1 -> MATLAB Function1/17(Izz)
  Constant4/1 -> MATLAB Function1/16(Iyy)
  p/1 -> MATLAB Function1/9(p)
  prop2body Matrix/1(R3to1) -> Moment Transform/1, Force Transform/1
  Moment Transform/1 -> Display1/1, Add/2
  Prop radius/1 -> prop behaviour/5(R)
  Gamma reference/1 -> PushPullDynamics/1(Gamma reference)
  qdot/1 -> MATLAB Function1/13(qdot)
  Constant1/1 -> prop behaviour/3(Cq)
  Throttle reference/1 -> Motor+ESC Dynamic/1(Throttle reference)
  3x3 Cross Product/1 -> Add/1
  q/1 -> MATLAB Function1/10(q)
  Density/1 -> prop behaviour/4(rho)
  Motor+ESC Dynamic/1(Omega) -> MATLAB Function1/7(omega), prop behaviour/1(Omega)
  ServoBlockDynamics/3(Etadotdot) -> MATLAB Function1/3(etadotdot)
  prop behaviour/2(M) -> Moment Transform/2
  Constant3/1 -> MATLAB Function1/15(Ixx)
  PushPullDynamics/1(Gamma) -> Bus Creator/2, MATLAB Function1/4(gamma), prop2body Matrix/2(gamma)  "gamma2"
  Constant2/1 -> 3x3 Cross Product/1
  Force Transform/1 -> F/1, 3x3 Cross Product/2
  MATLAB Function1/1(M) -> Display/1, Add/3
  ServoBlockDynamics/1(Eta) -> Bus Creator/1, MATLAB Function1/1(eta), prop2body Matrix/1(eta)  "eta2"
  r/1 -> MATLAB Function1/11(r)
  rdot/1 -> MATLAB Function1/14(rdot)
  Eta reference/1 -> ServoBlockDynamics/1(Eta reference)
  Bus Creator/1 -> TiltAngle/1
  PushPullDynamics/2(Gammadot) -> MATLAB Function1/5(gammadot)
  pdot/1 -> MATLAB Function1/12(pdot)
  prop behaviour/1(F) -> Force Transform/2
  Constant/1 -> prop behaviour/2(Ct)
  Add/1 -> M/1
  ServoBlockDynamics/2(Etadot) -> MATLAB Function1/2(etadot)

== system SimulinkOminidirectinalDrone/Vehicle Dynamic/actuator/Arm 3/STANDARD ARM MODEL CLOCKWISE/Motor+ESC Dynamic ==
  Throttle reference : Inport
  Derivative : Derivative
  G Motor : TransferFcn  Numerator=[9.19]  Denominator=[0.16 1]
  Transport Delay : TransportDelay  DelayTime=0.035
  Omega : Outport
  Omegadot : Outport  Port=2
  wires:
  Throttle reference/1 -> G Motor/1
  Derivative/1 -> Omegadot/1
  G Motor/1 -> Omega/1, Derivative/1

== system SimulinkOminidirectinalDrone/Vehicle Dynamic/actuator/Arm 3/STANDARD ARM MODEL CLOCKWISE/PushPullDynamics ==
  Gamma reference : Inport
  Derivative : Derivative
  Derivative1 : Derivative
  G pushpull : TransferFcn  Numerator=[1212.73]  Denominator=[1 51.105 1212.73]
  Saturation : Saturate  UpperLimit=pi/9  LowerLimit=-pi/9
  Saturation1 : Saturate  UpperLimit=pi/9  LowerLimit=-pi/9
  Gamma : Outport
  Gammadot : Outport  Port=2
  Gammadotdot : Outport  Port=3
  wires:
  Derivative/1 -> Gammadot/1, Derivative1/1
  Derivative1/1 -> Gammadotdot/1
  Gamma reference/1 -> Saturation/1
  G pushpull/1 -> Saturation1/1, Derivative/1
  Saturation/1 -> G pushpull/1
  Saturation1/1 -> Gamma/1

== system SimulinkOminidirectinalDrone/Vehicle Dynamic/actuator/Arm 3/STANDARD ARM MODEL CLOCKWISE/ServoBlockDynamics ==
  Eta reference : Inport
  Derivative : Derivative
  Derivative1 : Derivative
  G Servoblock : TransferFcn  Numerator=[1228.05]  Denominator=[1 49.1806 1228.05]
  Saturation : Saturate  UpperLimit=pi/9  LowerLimit=-pi/9
  Saturation1 : Saturate  UpperLimit=pi/9  LowerLimit=-pi/9
  Eta : Outport
  Etadot : Outport  Port=2
  Etadotdot : Outport  Port=3
  wires:
  Derivative/1 -> Etadot/1, Derivative1/1
  Derivative1/1 -> Etadotdot/1
  Eta reference/1 -> Saturation/1
  G Servoblock/1 -> Saturation1/1, Derivative/1
  Saturation/1 -> G Servoblock/1
  Saturation1/1 -> Eta/1

== system SimulinkOminidirectinalDrone/Vehicle Dynamic/actuator/Arm 4/STANDARD ARM MODEL CLOCKWISE/Motor+ESC Dynamic ==
  Throttle reference : Inport
  Derivative : Derivative
  G Motor : TransferFcn  Numerator=[9.19]  Denominator=[0.16 1]
  Transport Delay : TransportDelay  DelayTime=0.035
  Omega : Outport
  Omegadot : Outport  Port=2
  wires:
  Throttle reference/1 -> G Motor/1
  Derivative/1 -> Omegadot/1
  G Motor/1 -> Omega/1, Derivative/1

== system SimulinkOminidirectinalDrone/Vehicle Dynamic/actuator/Arm 4/STANDARD ARM MODEL CLOCKWISE/PushPullDynamics ==
  Gamma reference : Inport
  Derivative : Derivative
  Derivative1 : Derivative
  G pushpull : TransferFcn  Numerator=[1212.73]  Denominator=[1 51.105 1212.73]
  Saturation : Saturate  UpperLimit=pi/9  LowerLimit=-pi/9
  Saturation1 : Saturate  UpperLimit=pi/9  LowerLimit=-pi/9
  Gamma : Outport
  Gammadot : Outport  Port=2
  Gammadotdot : Outport  Port=3
  wires:
  Derivative/1 -> Gammadot/1, Derivative1/1
  Derivative1/1 -> Gammadotdot/1
  Gamma reference/1 -> Saturation/1
  G pushpull/1 -> Saturation1/1, Derivative/1
  Saturation/1 -> G pushpull/1
  Saturation1/1 -> Gamma/1

== system SimulinkOminidirectinalDrone/Vehicle Dynamic/actuator/Arm 4/STANDARD ARM MODEL CLOCKWISE/ServoBlockDynamics ==
  Eta reference : Inport
  Derivative : Derivative
  Derivative1 : Derivative
  G Servoblock : TransferFcn  Numerator=[1228.05]  Denominator=[1 49.1806 1228.05]
  Saturation : Saturate  UpperLimit=pi/9  LowerLimit=-pi/9
  Saturation1 : Saturate  UpperLimit=pi/9  LowerLimit=-pi/9
  Eta : Outport
  Etadot : Outport  Port=2
  Etadotdot : Outport  Port=3
  wires:
  Derivative/1 -> Etadot/1, Derivative1/1
  Derivative1/1 -> Etadotdot/1
  Eta reference/1 -> G Servoblock/1
  G Servoblock/1 -> Saturation1/1, Derivative/1
  Saturation1/1 -> Eta/1

== system SimulinkOminidirectinalDrone/Vehicle Dynamic/actuator/Arm1/STANDARD ARM MODEL CLOCKWISE/Motor+ESC Dynamic ==
  Throttle reference : Inport
  Derivative : Derivative
  G Motor : TransferFcn  Numerator=[9.19]  Denominator=[0.16 1]
  Gain : Gain  Gain=-1
  Gain1 : Gain  Gain=-1
  Transport Delay : TransportDelay  DelayTime=0.035
  Omega : Outport
  Omegadot : Outport  Port=2
  wires:
  Throttle reference/1 -> G Motor/1
  G Motor/1 -> Transport Delay/1
  Derivative/1 -> Gain1/1
  Transport Delay/1 -> Gain/1, Derivative/1
  Gain/1 -> Omega/1
  Gain1/1 -> Omegadot/1

== system SimulinkOminidirectinalDrone/Vehicle Dynamic/actuator/Arm1/STANDARD ARM MODEL CLOCKWISE/PushPullDynamics ==
  Gamma reference : Inport
  Derivative : Derivative
  Derivative1 : Derivative
  G pushpull : TransferFcn  Numerator=[1212.73]  Denominator=[1 51.105 1212.73]
  Saturation : Saturate  UpperLimit=pi/9  LowerLimit=-pi/9
  Saturation1 : Saturate  UpperLimit=pi/9  LowerLimit=-pi/9
  Gamma : Outport
  Gammadot : Outport  Port=2
  Gammadotdot : Outport  Port=3
  wires:
  Derivative/1 -> Gammadot/1, Derivative1/1
  Derivative1/1 -> Gammadotdot/1
  Gamma reference/1 -> Saturation/1
  G pushpull/1 -> Saturation1/1, Derivative/1
  Saturation/1 -> G pushpull/1
  Saturation1/1 -> Gamma/1

== system SimulinkOminidirectinalDrone/Vehicle Dynamic/actuator/Arm1/STANDARD ARM MODEL CLOCKWISE/ServoBlockDynamics ==
  Eta reference : Inport
  Derivative : Derivative
  Derivative1 : Derivative
  G Servoblock : TransferFcn  Numerator=[1228.05]  Denominator=[1 49.1806 1228.05]
  Saturation : Saturate  UpperLimit=pi/9  LowerLimit=-pi/9
  Saturation1 : Saturate  UpperLimit=pi/9  LowerLimit=-pi/9
  Eta : Outport
  Etadot : Outport  Port=2
  Etadotdot : Outport  Port=3
  wires:
  Derivative/1 -> Etadot/1, Derivative1/1
  Derivative1/1 -> Etadotdot/1
  Eta reference/1 -> Saturation/1
  G Servoblock/1 -> Saturation1/1, Derivative/1
  Saturation/1 -> G Servoblock/1
  Saturation1/1 -> Eta/1

== system SimulinkOminidirectinalDrone/Vehicle Dynamic/actuator/Arm2/STANDARD ARM MODEL CLOCKWISE/Motor+ESC Dynamic ==
  Throttle reference : Inport
  Derivative : Derivative
  G Motor : TransferFcn  Numerator=[9.19]  Denominator=[0.16 1]
  Gain : Gain  Gain=-1
  Gain1 : Gain  Gain=-1
  Transport Delay : TransportDelay  DelayTime=0.035
  Omega : Outport
  Omegadot : Outport  Port=2
  wires:
  Throttle reference/1 -> G Motor/1
  G Motor/1 -> Transport Delay/1
  Transport Delay/1 -> Gain/1, Derivative/1
  Derivative/1 -> Gain1/1
  Gain/1 -> Omega/1
  Gain1/1 -> Omegadot/1

== system SimulinkOminidirectinalDrone/Vehicle Dynamic/actuator/Arm2/STANDARD ARM MODEL CLOCKWISE/PushPullDynamics ==
  Gamma reference : Inport
  Derivative : Derivative
  Derivative1 : Derivative
  G pushpull : TransferFcn  Numerator=[1212.73]  Denominator=[1 51.105 1212.73]
  Saturation1 : Saturate  UpperLimit=pi/9  LowerLimit=-pi/9
  Saturation2 : Saturate  UpperLimit=pi/9  LowerLimit=-pi/9
  Gamma : Outport
  Gammadot : Outport  Port=2
  Gammadotdot : Outport  Port=3
  wires:
  Derivative/1 -> Gammadot/1, Derivative1/1
  Derivative1/1 -> Gammadotdot/1
  G pushpull/1 -> Saturation1/1, Derivative/1
  Gamma reference/1 -> Saturation2/1
  Saturation1/1 -> Gamma/1
  Saturation2/1 -> G pushpull/1

== system SimulinkOminidirectinalDrone/Vehicle Dynamic/actuator/Arm2/STANDARD ARM MODEL CLOCKWISE/ServoBlockDynamics ==
  Eta reference : Inport
  Derivative : Derivative
  Derivative1 : Derivative
  G Servoblock : TransferFcn  Numerator=[1228.05]  Denominator=[1 49.1806 1228.05]
  Saturation1 : Saturate  UpperLimit=pi/9  LowerLimit=-pi/9
  Saturation2 : Saturate  UpperLimit=pi/9  LowerLimit=-pi/9
  Eta : Outport
  Etadot : Outport  Port=2
  Etadotdot : Outport  Port=3
  wires:
  Derivative/1 -> Etadot/1, Derivative1/1
  Derivative1/1 -> Etadotdot/1
  G Servoblock/1 -> Saturation1/1, Derivative/1
  Eta reference/1 -> Saturation2/1
  Saturation1/1 -> Eta/1
  Saturation2/1 -> G Servoblock/1

== matlab function SimulinkOminidirectinalDrone/Vehicle Dynamic/actuator/Arm 3/STANDARD ARM MODEL CLOCKWISE/prop2body Matrix ==
  data: eta input; R3to1 output; gamma input
function R3to1 = prop2body(eta, gamma)
%#codegen
% Input: eta, gamma
% Output: R3to1 (3x3 rotation matrix)

R3to1 = [ cos(eta),            sin(gamma)*sin(eta),   cos(gamma)*sin(eta);
          0,                   cos(gamma),            -sin(gamma);
         -sin(eta),            cos(eta)*sin(gamma),   cos(gamma)*cos(eta) ];
end

== matlab function SimulinkOminidirectinalDrone/Vehicle Dynamic/actuator/Arm 4/STANDARD ARM MODEL CLOCKWISE/MATLAB Function1 ==
  data: eta input; M output; etadot input; etadotdot input; gamma input; gammadot input; gammadotdot input; omega input; omegadot input; p input; q input; r input; pdot input; qdot input; rdot input; Ixx input; Iyy input; Izz input
function M = fcn(eta,etadot,etadotdot,gamma,gammadot,gammadotdot,omega,omegadot, p,q,r,pdot,qdot,rdot,Ixx,Iyy,Izz)

M1reactX = (1/4)*(-2*Ixx*q*r+Iyy*q*r+Izz*q*r+3*Iyy*cos(2*gamma)*q*r-3*cos(2*gamma)*q*r-...
    4*Izz*sin(gamma)*omega*r+2*Iyy*etadot*r+2*Izz*etadot+2*Iyy*cos(2*gamma)*etadot*r-2*Izz*cos(2*gamma)*etadot*r-2*Ixx*pdot-Iyy*pdot...
    -Izz*pdot+Iyy*cos(2*gamma)*pdot-Izz*cos(2*gamma)*pdot-2*Iyy*p*sin(2*gamma)*gammadot+2*Izz*p*sin(2*gamma)*gammadot...
    -sin(2*eta)*(4*(Ixx-Iyy)*p*sin(gamma)*omega+2*(Iyy-Izz)*r*sin(2*gamma)*gammadot-(2*Ixx-Iyy-Izz)*(rdot+p*(q+2*etadot))...
    -(Iyy-Izz)*cos(2*eta)*(rdot+p*(q+2*etadot)))-cos(2*eta)*(4*(Ixx-Iyy)*r*sin(gamma)*omega+2*(Izz-Iyy)*p*sin(2*gamma)*gammadot...
    +(2*Ixx-Iyy-Izz)*(pdot-r*(q+2*etadot))+(Iyy-Izz)*cos(2*gamma)*(pdot-r*(q+2*etadot)))...
    -2*cos(eta)*(2*(Ixx-Iyy+Izz)*cos(gamma)*omega*(q+etadot)+(Iyy-Izz)*sin(2*gamma)*(q-r+etadot)*...
    (q+r+etadot)+2*Ixx*gammadotdot)-2*sin(eta)*(-2*(-Ixx+Iyy+Izz)*sin(gamma)*omega*gammadot-2*Ixx*(q+etadot)*gammadot+2*(Iyy-Izz)*...
    cos(2*gamma)*(q+etadot)*gammadot+2*Izz*cos(gamma)*omegadot-(Iyy-Izz)*sin(2*gamma)*(p*r-qdot-etadotdot)));

M1reactY = (1/4)*(-2*Ixx*sin(2*eta)*p^2+Iyy*sin(2*eta)*p^2+Izz*sin(2*eta)*p^2-4*Ixx*cos(2*eta)*r*p+...
    2*Iyy*cos(2*eta)*r*p+2*Izz*cos(2*eta)*r*p-4*Ixx*sin(eta)*gammadot*p+2*Ixx*r^2*sin(2*eta)-...
    Iyy*r^2*sin(2*eta)-Izz*r^2*sin(2*eta)-2*Iyy*qdot-2*Izz*qdot-4*Ixx*cos(eta)*r*gammadot-4*(Ixx-Iyy-Izz)*cos(gamma)*omega*(cos(eta)*p...
    -r*sin(eta)+gammadot)+2*(Iyy-Izz)*sin(2*gamma)*(-sin(eta)*(q*r+pdot)+cos(eta)*(p*q-rdot)+2*gammadot*(q+etadot))+4*Izz*sin(gamma)*...
    omegadot-2*Iyy*etadotdot-2*Izz*etadotdot-2*(Iyy-Izz)*cos(2*gamma)*(qdot+(cos(eta)*r+p*sin(eta))*(cos(eta)*p-r*sin(eta)+2*gammadot)+etadotdot));

M1reactZ = (1/4)*(-2*(Iyy-Izz)*sin(2*gamma)*sin(eta)*p^2-(4*(Iyy-Izz)*cos(2*gamma)*etadot*(sin(eta)^2+...
    (2*(-2*Ixx+Iyy+Izz)*(cos(eta)^2)-(Iyy-Izz)*cos(2*gamma)*(cos(2*eta)-3))*q...
    -4*(Izz+(Iyy-Ixx)*cos(2*eta))*sin(gamma)*omega+2*(Iyy-Izz)*cos(eta)*sin(2*gamma)*(r+2*sin(eta)*gammadot)+...
    2*(Iyy+Izz+(-2*Ixx+Iyy+Izz)*cos(2*eta))*etadot)*p-2*Ixx*rdot-Iyy*rdot-Izz*rdot+Iyy*cos(2*gamma)*...
    rdot-Izz*cos(2*gamma)*rdot-2*Iyy*r*sin(2*gamma)*gammadot+2*Izz*r*sin(2*gamma)*gammadot-cos(2*gamma)*((-2*Ixx+Iyy+Izz+(Izz-Iyy)*cos(2*gamma))*rdot+...
    2*(Iyy-Izz)*r*sin(2*gamma)*gammadot)-sin(2*eta)*(4*(Iyy-Ixx)*r*sin(gamma)*omega+(2*Ixx-Iyy-Izz)*(r*(q+2*etadot)-pdot)...
    +(Iyy-Izz)*cos(2*gamma)*(r*(q+2*etadot)-pdot))-2*sin(eta)*(-(Iyy-Izz)*sin(2*gamma)*(q+etadot)^2 ...
    -2*(Ixx-Iyy+Izz)*cos(gamma)*omega*(q+etadot)-2*Ixx*gammadotdot)-2*cos(eta)*(-2*(-Ixx+Iyy+Izz)*sin(gamma)*omega*gammadot...
    -2*Ixx*(q+etadot)*gammadot)+2*(Iyy-Izz)*cos(2*gamma)*(q+etadot)*gammadot+2*Izz*cos(gamma)*omegadot+(Iyy-Izz)*sin(2*gamma)*(qdot+etadotdot)));

M = [ M1reactX;
      M1reactY;
      M1reactZ];

== matlab function SimulinkOminidirectinalDrone/Vehicle Dynamic/actuator/Arm 4/STANDARD ARM MODEL CLOCKWISE/prop behaviour ==
  data: Omega input; Ct input; Cq input; rho input; F output; R input; M output
function [F, M] = fcn(Omega, Ct, Cq, rho, R)
%#codegen
% Inputs:
%   rho   - air density (kg/m^3)
%   R     - propeller radius (m)
%   Omega - angular velocity (rad/s)
%   Ct    - thrust coefficient
%   Cq    - torque coefficient
%
% Outputs:
%   T - Thrust force (N)
%   Q - Torque (Nm)
% Rotor disk area
A = pi * R^2;
% Thrust (eq. 4.38)
F = [0; 0; rho * A * (Omega * R)^2 * Ct];
% Torque (eq. 4.39)
M = [0; 0; rho * A * (Omega * R)^2 * R * Cq];


end

== matlab function SimulinkOminidirectinalDrone/Vehicle Dynamic/actuator/Arm 4/STANDARD ARM MODEL CLOCKWISE/prop2body Matrix ==
  data: eta input; R3to1 output; gamma input
function R3to1 = prop2body(eta, gamma)
%#codegen
% Input: eta, gamma
% Output: R3to1 (3x3 rotation matrix)

R3to1 = [ cos(eta),            sin(gamma)*sin(eta),   cos(gamma)*sin(eta);
          0,                   cos(gamma),            -sin(gamma);
         -sin(eta),            cos(eta)*sin(gamma),   cos(gamma)*cos(eta) ];
end

== matlab function SimulinkOminidirectinalDrone/Vehicle Dynamic/actuator/Arm1/STANDARD ARM MODEL CLOCKWISE/MATLAB Function1 ==
  data: eta input; M output; etadot input; etadotdot input; gamma input; gammadot input; gammadotdot input; omega input; omegadot input; p input; q input; r input; pdot input; qdot input; rdot input; Ixx input; Iyy input; Izz input
function M = fcn(eta,etadot,etadotdot,gamma,gammadot,gammadotdot,omega,omegadot, p,q,r,pdot,qdot,rdot,Ixx,Iyy,Izz)

M1reactX = (1/4)*(-2*Ixx*q*r+Iyy*q*r+Izz*q*r+3*Iyy*cos(2*gamma)*q*r-3*cos(2*gamma)*q*r-...
    4*Izz*sin(gamma)*omega*r+2*Iyy*etadot*r+2*Izz*etadot+2*Iyy*cos(2*gamma)*etadot*r-2*Izz*cos(2*gamma)*etadot*r-2*Ixx*pdot-Iyy*pdot...
    -Izz*pdot+Iyy*cos(2*gamma)*pdot-Izz*cos(2*gamma)*pdot-2*Iyy*p*sin(2*gamma)*gammadot+2*Izz*p*sin(2*gamma)*gammadot...
    -sin(2*eta)*(4*(Ixx-Iyy)*p*sin(gamma)*omega+2*(Iyy-Izz)*r*sin(2*gamma)*gammadot-(2*Ixx-Iyy-Izz)*(rdot+p*(q+2*etadot))...
    -(Iyy-Izz)*cos(2*eta)*(rdot+p*(q+2*etadot)))-cos(2*eta)*(4*(Ixx-Iyy)*r*sin(gamma)*omega+2*(Izz-Iyy)*p*sin(2*gamma)*gammadot...
    +(2*Ixx-Iyy-Izz)*(pdot-r*(q+2*etadot))+(Iyy-Izz)*cos(2*gamma)*(pdot-r*(q+2*etadot)))...
    -2*cos(eta)*(2*(Ixx-Iyy+Izz)*cos(gamma)*omega*(q+etadot)+(Iyy-Izz)*sin(2*gamma)*(q-r+etadot)*...
    (q+r+etadot)+2*Ixx*gammadotdot)-2*sin(eta)*(-2*(-Ixx+Iyy+Izz)*sin(gamma)*omega*gammadot-2*Ixx*(q+etadot)*gammadot+2*(Iyy-Izz)*...
    cos(2*gamma)*(q+etadot)*gammadot+2*Izz*cos(gamma)*omegadot-(Iyy-Izz)*sin(2*gamma)*(p*r-qdot-etadotdot)));

M1reactY = (1/4)*(-2*Ixx*sin(2*eta)*p^2+Iyy*sin(2*eta)*p^2+Izz*sin(2*eta)*p^2-4*Ixx*cos(2*eta)*r*p+...
    2*Iyy*cos(2*eta)*r*p+2*Izz*cos(2*eta)*r*p-4*Ixx*sin(eta)*gammadot*p+2*Ixx*r^2*sin(2*eta)-...
    Iyy*r^2*sin(2*eta)-Izz*r^2*sin(2*eta)-2*Iyy*qdot-2*Izz*qdot-4*Ixx*cos(eta)*r*gammadot-4*(Ixx-Iyy-Izz)*cos(gamma)*omega*(cos(eta)*p...
    -r*sin(eta)+gammadot)+2*(Iyy-Izz)*sin(2*gamma)*(-sin(eta)*(q*r+pdot)+cos(eta)*(p*q-rdot)+2*gammadot*(q+etadot))+4*Izz*sin(gamma)*...
    omegadot-2*Iyy*etadotdot-2*Izz*etadotdot-2*(Iyy-Izz)*cos(2*gamma)*(qdot+(cos(eta)*r+p*sin(eta))*(cos(eta)*p-r*sin(eta)+2*gammadot)+etadotdot));

M1reactZ = (1/4)*(-2*(Iyy-Izz)*sin(2*gamma)*sin(eta)*p^2-(4*(Iyy-Izz)*cos(2*gamma)*etadot*(sin(eta)^2+...
    (2*(-2*Ixx+Iyy+Izz)*(cos(eta)^2)-(Iyy-Izz)*cos(2*gamma)*(cos(2*eta)-3))*q...
    -4*(Izz+(Iyy-Ixx)*cos(2*eta))*sin(gamma)*omega+2*(Iyy-Izz)*cos(eta)*sin(2*gamma)*(r+2*sin(eta)*gammadot)+...
    2*(Iyy+Izz+(-2*Ixx+Iyy+Izz)*cos(2*eta))*etadot)*p-2*Ixx*rdot-Iyy*rdot-Izz*rdot+Iyy*cos(2*gamma)*...
    rdot-Izz*cos(2*gamma)*rdot-2*Iyy*r*sin(2*gamma)*gammadot+2*Izz*r*sin(2*gamma)*gammadot-cos(2*gamma)*((-2*Ixx+Iyy+Izz+(Izz-Iyy)*cos(2*gamma))*rdot+...
    2*(Iyy-Izz)*r*sin(2*gamma)*gammadot)-sin(2*eta)*(4*(Iyy-Ixx)*r*sin(gamma)*omega+(2*Ixx-Iyy-Izz)*(r*(q+2*etadot)-pdot)...
    +(Iyy-Izz)*cos(2*gamma)*(r*(q+2*etadot)-pdot))-2*sin(eta)*(-(Iyy-Izz)*sin(2*gamma)*(q+etadot)^2 ...
    -2*(Ixx-Iyy+Izz)*cos(gamma)*omega*(q+etadot)-2*Ixx*gammadotdot)-2*cos(eta)*(-2*(-Ixx+Iyy+Izz)*sin(gamma)*omega*gammadot...
    -2*Ixx*(q+etadot)*gammadot)+2*(Iyy-Izz)*cos(2*gamma)*(q+etadot)*gammadot+2*Izz*cos(gamma)*omegadot+(Iyy-Izz)*sin(2*gamma)*(qdot+etadotdot)));

M = [ M1reactX;
      M1reactY;
      M1reactZ];

== matlab function SimulinkOminidirectinalDrone/Vehicle Dynamic/actuator/Arm1/STANDARD ARM MODEL CLOCKWISE/prop behaviour ==
  data: Omega input; Ct input; Cq input; rho input; F output; R input; M output
function [F, M] = fcn(Omega, Ct, Cq, rho, R)
%#codegen
% Inputs:
%   rho   - air density (kg/m^3)
%   R     - propeller radius (m)
%   Omega - angular velocity (rad/s)
%   Ct    - thrust coefficient
%   Cq    - torque coefficient
%
% Outputs:
%   T - Thrust force (N)
%   Q - Torque (Nm)
% Rotor disk area
A = pi * R^2;
% Thrust (eq. 4.38)
F = [0; 0; rho * A * (Omega * R)^2 * Ct];
% Torque (eq. 4.39)
M = [0; 0; rho * A * (Omega * R)^2 * R * Cq];

end

== matlab function SimulinkOminidirectinalDrone/Vehicle Dynamic/actuator/Arm1/STANDARD ARM MODEL CLOCKWISE/prop2body Matrix ==
  data: eta input; R3to1 output; gamma input
function R3to1 = prop2body(eta, gamma)
%#codegen
% Input: eta, gamma
% Output: R3to1 (3x3 rotation matrix)

R3to1 = [ cos(eta),            sin(gamma)*sin(eta),   cos(gamma)*sin(eta);
          0,                   cos(gamma),            -sin(gamma);
         -sin(eta),            cos(eta)*sin(gamma),   cos(gamma)*cos(eta) ];
end

== matlab function SimulinkOminidirectinalDrone/Subsystem/MATLAB Function ==
  data: B output
function B = compute_B_matrix()
    % Tham số từ luận văn (ước lượng, cần điều chỉnh theo thực tế)
    mu = 0.0001;        % Hệ số thrust
    kappa = 0.001;      % Hệ số torque
    J = 110.9e-6;       % Moment quán tính (kg·m²)
    Omega = 100;        % Tốc độ quay propeller (rad/s)
    tr = 0.1;           % Rise time servo (s)
    L = 0.25;           % Chiều dài arm (m)
    H = 0.05;           % Chiều cao hub (m)
    T0 = 1.5;           % Thrust tại hover (N)

    % Submatrix cho Standard Arm (4x3)
    B_std = [-L*mu, -J*Omega/tr, H*T0;
             H*T0, L*T0, J*Omega/tr;
             kappa, 0, 0;
             mu, 0, 0];

    % Ma trận B đầy đủ (4x12) cho 4 arms
    % Arm 1, 2, 3, 4 với rotation và dấu ± cho kappa
    B = zeros(4, 12);
    % Arm 1 (Standard)
    B(:, 1:3) = B_std;
    % Arm 2 (Rotate 90 deg, ví dụ: đảo dấu ở hàng 1, 2)
    B(:, 4:6) = [-H*T0, -L*T0, J*Omega/tr;
                 -L*mu, -J*Omega/tr, 0;
                 kappa, 0, 0;
                 mu, 0, 0];
    % Arm 3 (Rotate 180 deg, ví dụ: đảo dấu)
    B(:, 7:9) = [L*mu, J*Omega/tr, H*T0;
                 -H*T0, -L*T0, J*Omega/tr;
                 kappa, 0, 0;
                 mu, 0, 0];
    % Arm 4 (Rotate 270 deg)
    B(:, 10:12) = [H*T0, L*T0, -J*Omega/tr;
                   L*mu, J*Omega/tr, 0;
                   -kappa, 0, 0;
                   mu, 0, 0];
end

== matlab function SimulinkOminidirectinalDrone/Subsystem/MATLAB Function1 ==
  data: v input; u output; B input; W input
function u = weighted_pseudoinverse_allocator(v, B, W)
    % Input: v (4x1), B (4x12), W (12x12 diagonal)
    % Output: u (12x1)
    
    % Tính weighted pseudoinverse
    % Winv = inv(W); % Ma trận nghịch đảo trọng số
    u = W \ B' * ((B / W * B') \ v);
end

== matlab function SimulinkOminidirectinalDrone/Vehicle Dynamic/actuator/Arm2/STANDARD ARM MODEL CLOCKWISE/prop behaviour ==
  data: Omega input; Ct input; Cq input; rho input; F output; R input; M output
function [F, M] = fcn(Omega, Ct, Cq, rho, R)
%#codegen
% Inputs:
%   rho   - air density (kg/m^3)
%   R     - propeller radius (m)
%   Omega - angular velocity (rad/s)
%   Ct    - thrust coefficient
%   Cq    - torque coefficient
%
% Outputs:
%   T - Thrust force (N)
%   Q - Torque (Nm)
% Rotor disk area
A = pi * R^2;
% Thrust (eq. 4.38)
F = [0; 0; rho * A * (Omega * R)^2 * Ct];
% Torque (eq. 4.39)
M = [0; 0; rho * A * (Omega * R)^2 * R * Cq];

end

== matlab function SimulinkOminidirectinalDrone/Vehicle Dynamic/actuator/Arm2/STANDARD ARM MODEL CLOCKWISE/prop2body Matrix ==
  data: eta input; R3to1 output; gamma input
function R3to1 = prop2body(eta, gamma)
%#codegen
% Input: eta, gamma
% Output: R3to1 (3x3 rotation matrix)

R3to1 = [ cos(eta),            sin(gamma)*sin(eta),   cos(gamma)*sin(eta);
          0,                   cos(gamma),            -sin(gamma);
         -sin(eta),            cos(eta)*sin(gamma),   cos(gamma)*cos(eta) ];
end
